simulink model "chopper"  (R2021a)
settings: Solver=VariableStepAuto  StartTime=0.0  StopTime=inf  RelTol=1e-3
libraries: spsCurrentMeasurementLib x2, spsDCVoltageSourceLib x2, spsIGBTLib x2, spsSeriesRLCBranchLib x2, spsVoltageMeasurementLib x2, spsDiodeLib x1, spspowerguiLib x1
settings Model: Creator=User  LastModifiedBy=User

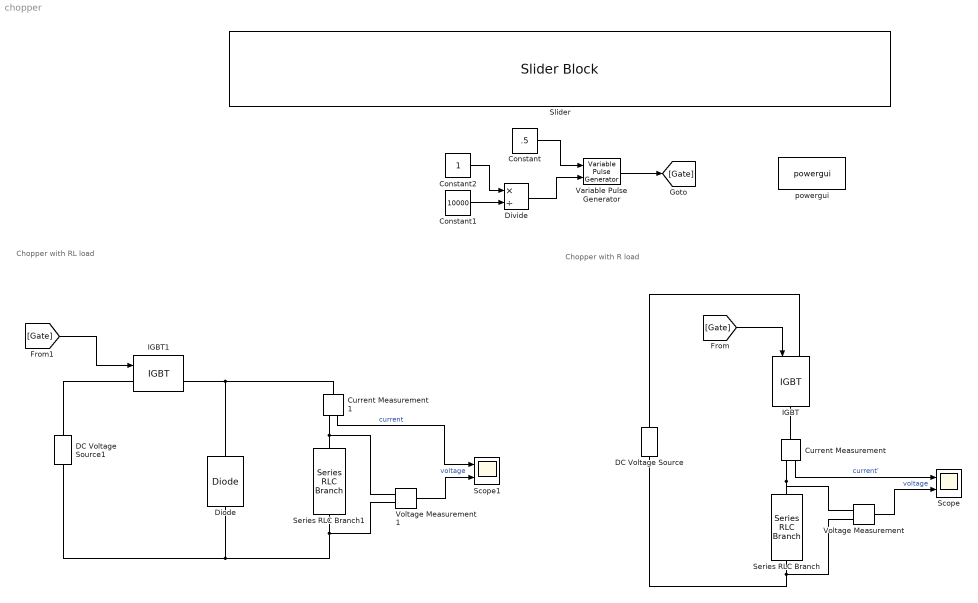
== system chopper ==
  note: Chopper with RL load
  note: Chopper with R load
  Constant : Constant  Value=.5
  Constant1 : Constant  Value=10000
  Constant2 : Constant
  Current Measurement : spsCurrentMeasurementLib/Current Measurement  PhasorSimulation=off  OutputType=Complex  PSBequivalent=0
  Current Measurement1 : spsCurrentMeasurementLib/Current Measurement  PhasorSimulation=off  OutputType=Complex  PSBequivalent=0
  DC Voltage Source : spsDCVoltageSourceLib/DC Voltage Source  Amplitude=100  Measurements=None
  DC Voltage Source1 : spsDCVoltageSourceLib/DC Voltage Source  Amplitude=100  Measurements=None
  Diode : spsDiodeLib/Diode  Ron=0.001  Lon=0  Vf=0.8  IC=0  UseSnubber=0  Rs=500  Cs=250e-9  Measurements=off
  Divide : Product  Inputs=*/
  IGBT : spsIGBTLib/IGBT  Ron=0.001  Lon=0  Vf=1  Tf=1e-6  Tt=2e-6  IC=0  Rs=1e5  Cs=inf  Measurements=off
  IGBT1 : spsIGBTLib/IGBT  Ron=0.001  Lon=0  Vf=1  Tf=1e-6  Tt=2e-6  IC=0  Rs=1e5  Cs=inf  Measurements=on
  Scope : Scope  NumInputPorts=2
  Scope1 : Scope  NumInputPorts=2
  Series RLC Branch : spsSeriesRLCBranchLib/Series RLC Branch  LConnTagsString=__new0  RConnTagsString=__new0  BranchType=R  Resistance=10  Inductance=1e-3  SetiL0=off  InitialCurrent=0  Capacitance=1e-6  Setx0=off  InitialVoltage=0  Measurements=None
  Series RLC Branch1 : spsSeriesRLCBranchLib/Series RLC Branch  LConnTagsString=__new0  RConnTagsString=__new0  BranchType=RL  Resistance=10  Inductance=1e-3  SetiL0=off  InitialCurrent=0  Capacitance=1e-6  Setx0=off  InitialVoltage=0  Measurements=None
  Slider : SliderBlock  ScaleMin=50  ScaleMax=10000  TickInterval=500
  Variable Pulse Generator : VariablePulseGenerator  SampleTime=0.1
  Voltage Measurement : spsVoltageMeasurementLib/Voltage Measurement  PhasorSimulation=off  OutputType=Complex  PSBequivalent=0
  Voltage Measurement1 : spsVoltageMeasurementLib/Voltage Measurement  PhasorSimulation=off  OutputType=Complex  PSBequivalent=0
  powergui : spspowerguiLib/powergui  Priority=1  SimulationMode=Continuous  SampleTime=50e-6  frequency=60  Iterations=50  frequencyindice=0  Pbase=100e6  ErrMax=1e-4  UnitsV=kV  UnitsW=MW  buscounter=0  FunctionMessages=off  echomessages=off  EnableUseOfTLC=off  CurrentSourceSwitches=off  DisableSnubberDevices=off  DisableRonSwitches=off  DisableVfSwitches=off  DisplayEquations=off  AutomaticDiscreteSolvers=off  SolverType=Tustin/Backward Euler (TBE)  Interpol=off  ExternalGateDelay=off  methode=off  Ts=100  x0status=blocks  SPID=on  SwTol=0  HookPort=off  NonlinearTolerance=1e-4  nMaxIteration=100  ContinueOnMaxIteration=off  RestoreLinks=warning  ResistiveCurrentMeasurement=off  Frange=[0:2:500]  Ylog=off  Xlog=on  ShowGrid=off  save=off  variable=ZData  structure=0  ZoomFFT=off  StartTime=0.0  cycles=1  DisplayStyle=1  fundamental=60  FreqAxis=off  MaxFrequency=1000  frequencyindicesteady=1  RmsSteady=1  display=off
  wires:
  [Gate] -> IGBT/1
  Voltage Measurement/1 -> Scope/2  "voltage"
  Current Measurement/1 -> Scope/1  "current'"
  Current Measurement1/1 -> Scope1/1  "current"
  Voltage Measurement1/1 -> Scope1/2  "voltage"
  [Gate] -> IGBT1/1
  Constant/1 -> Variable Pulse Generator/1
  Constant1/1 -> Divide/2
  Variable Pulse Generator/1 -> [Gate]
  Divide/1 -> Variable Pulse Generator/2
  Constant2/1 -> Divide/1
  connections:
  IGBT/RConn1 -- Current Measurement/LConn1
  DC Voltage Source/RConn1 -- IGBT/LConn1
  DC Voltage Source/LConn1 -- Voltage Measurement/LConn2 -- Series RLC Branch/RConn1
  Series RLC Branch/LConn1 -- Voltage Measurement/LConn1 -- Current Measurement/RConn1
  Voltage Measurement1/LConn2 -- Diode/LConn1 -- DC Voltage Source1/LConn1 -- Series RLC Branch1/RConn1
  Voltage Measurement1/LConn1 -- Series RLC Branch1/LConn1 -- Current Measurement1/RConn1
  DC Voltage Source1/RConn1 -- IGBT1/LConn1
  Current Measurement1/LConn1 -- Diode/RConn1 -- IGBT1/RConn1
